simulink library "ESTS_FRIC"  (R2024b)
settings: Solver=VariableStepAuto  StartTime=0.0  StopTime=10.0  RelTol=1e-3
libraries: ESTS_FRIC_HILO x1, ESTS_FRIC_SLIP x1
settings Model: Creator=blatak  LastModifiedBy=blatak
settings ModelReferenceCC: EnableRefExpFcnMdlSchedulingChecks=on
settings RTWCC: GPUComputeCapability=3.5

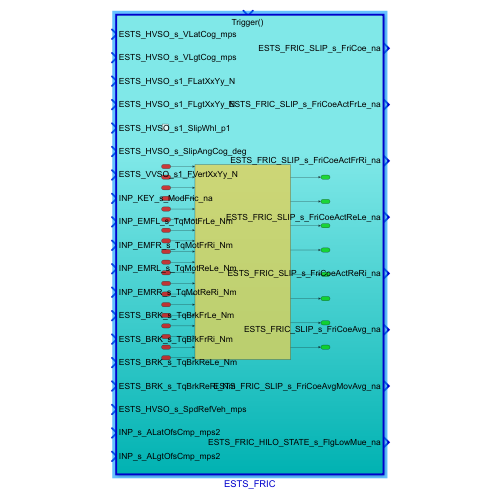
[thumbnail: Simulink's stored preview of the top-level diagram]
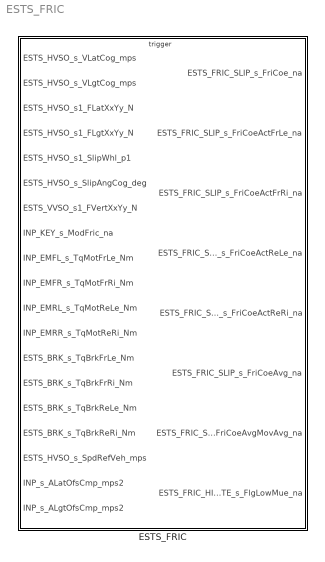
== system ESTS_FRIC ==
  ESTS_FRIC : Subsystem

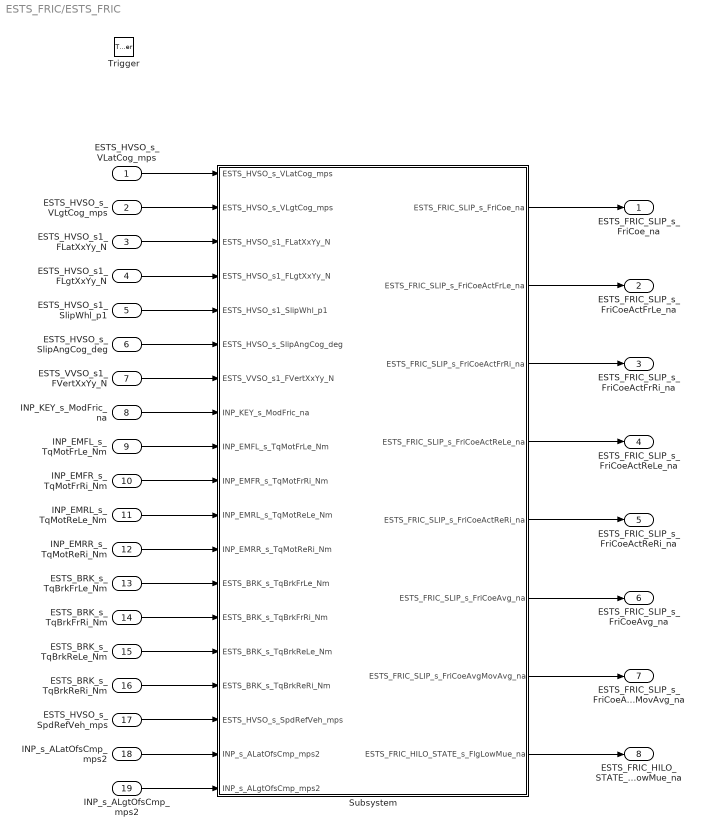
== system ESTS_FRIC/ESTS_FRIC ==
  ESTS_HVSO_s_VLatCog_mps : Inport
  ESTS_HVSO_s_VLgtCog_mps : Inport  Port=2
  ESTS_HVSO_s1_FLatXxYy_N : Inport  Port=3
  ESTS_HVSO_s1_FLgtXxYy_N : Inport  Port=4
  ESTS_HVSO_s1_SlipWhl_p1 : Inport  Port=5
  ESTS_HVSO_s_SlipAngCog_deg : Inport  Port=6
  ESTS_VVSO_s1_FVertXxYy_N : Inport  Port=7
  INP_KEY_s_ModFric_na : Inport  Port=8
  INP_EMFL_s_TqMotFrLe_Nm : Inport  Port=9
  INP_EMFR_s_TqMotFrRi_Nm : Inport  Port=10
  INP_EMRL_s_TqMotReLe_Nm : Inport  Port=11
  INP_EMRR_s_TqMotReRi_Nm : Inport  Port=12
  ESTS_BRK_s_TqBrkFrLe_Nm : Inport  Port=13
  ESTS_BRK_s_TqBrkFrRi_Nm : Inport  Port=14
  ESTS_BRK_s_TqBrkReLe_Nm : Inport  Port=15
  ESTS_BRK_s_TqBrkReRi_Nm : Inport  Port=16
  ESTS_HVSO_s_SpdRefVeh_mps : Inport  Port=17
  INP_s_ALatOfsCmp_mps2 : Inport  Port=18
  INP_s_ALgtOfsCmp_mps2 : Inport  Port=19
  Trigger : TriggerPort  TriggerType=function-call  VariantControl=(inherit)  PortDimensions=1
  Subsystem : Subsystem
  ESTS_FRIC_SLIP_s_FriCoe_na : Outport
  ESTS_FRIC_SLIP_s_FriCoeActFrLe_na : Outport  Port=2
  ESTS_FRIC_SLIP_s_FriCoeActFrRi_na : Outport  Port=3
  ESTS_FRIC_SLIP_s_FriCoeActReLe_na : Outport  Port=4
  ESTS_FRIC_SLIP_s_FriCoeActReRi_na : Outport  Port=5
  ESTS_FRIC_SLIP_s_FriCoeAvg_na : Outport  Port=6
  ESTS_FRIC_SLIP_s_FriCoeAvgMovAvg_na : Outport  Port=7
  ESTS_FRIC_HILO_STATE_s_FlgLowMue_na : Outport  Port=8
  wires:
  Subsystem/1(ESTS_FRIC_SLIP_s_FriCoe_na) -> ESTS_FRIC_SLIP_s_FriCoe_na/1
  Subsystem/2(ESTS_FRIC_SLIP_s_FriCoeActFrLe_na) -> ESTS_FRIC_SLIP_s_FriCoeActFrLe_na/1
  Subsystem/3(ESTS_FRIC_SLIP_s_FriCoeActFrRi_na) -> ESTS_FRIC_SLIP_s_FriCoeActFrRi_na/1
  Subsystem/4(ESTS_FRIC_SLIP_s_FriCoeActReLe_na) -> ESTS_FRIC_SLIP_s_FriCoeActReLe_na/1
  Subsystem/5(ESTS_FRIC_SLIP_s_FriCoeActReRi_na) -> ESTS_FRIC_SLIP_s_FriCoeActReRi_na/1
  Subsystem/6(ESTS_FRIC_SLIP_s_FriCoeAvg_na) -> ESTS_FRIC_SLIP_s_FriCoeAvg_na/1
  Subsystem/7(ESTS_FRIC_SLIP_s_FriCoeAvgMovAvg_na) -> ESTS_FRIC_SLIP_s_FriCoeAvgMovAvg_na/1
  Subsystem/8(ESTS_FRIC_HILO_STATE_s_FlgLowMue_na) -> ESTS_FRIC_HILO_STATE_s_FlgLowMue_na/1
  ESTS_HVSO_s_VLatCog_mps/1 -> Subsystem/1(ESTS_HVSO_s_VLatCog_mps)
  ESTS_HVSO_s_VLgtCog_mps/1 -> Subsystem/2(ESTS_HVSO_s_VLgtCog_mps)
  ESTS_HVSO_s1_FLatXxYy_N/1 -> Subsystem/3(ESTS_HVSO_s1_FLatXxYy_N)
  ESTS_HVSO_s1_FLgtXxYy_N/1 -> Subsystem/4(ESTS_HVSO_s1_FLgtXxYy_N)
  ESTS_HVSO_s1_SlipWhl_p1/1 -> Subsystem/5(ESTS_HVSO_s1_SlipWhl_p1)
  ESTS_HVSO_s_SlipAngCog_deg/1 -> Subsystem/6(ESTS_HVSO_s_SlipAngCog_deg)
  ESTS_VVSO_s1_FVertXxYy_N/1 -> Subsystem/7(ESTS_VVSO_s1_FVertXxYy_N)
  INP_KEY_s_ModFric_na/1 -> Subsystem/8(INP_KEY_s_ModFric_na)
  INP_EMFL_s_TqMotFrLe_Nm/1 -> Subsystem/9(INP_EMFL_s_TqMotFrLe_Nm)
  INP_EMFR_s_TqMotFrRi_Nm/1 -> Subsystem/10(INP_EMFR_s_TqMotFrRi_Nm)
  INP_EMRL_s_TqMotReLe_Nm/1 -> Subsystem/11(INP_EMRL_s_TqMotReLe_Nm)
  INP_EMRR_s_TqMotReRi_Nm/1 -> Subsystem/12(INP_EMRR_s_TqMotReRi_Nm)
  ESTS_BRK_s_TqBrkFrLe_Nm/1 -> Subsystem/13(ESTS_BRK_s_TqBrkFrLe_Nm)
  ESTS_BRK_s_TqBrkFrRi_Nm/1 -> Subsystem/14(ESTS_BRK_s_TqBrkFrRi_Nm)
  ESTS_BRK_s_TqBrkReLe_Nm/1 -> Subsystem/15(ESTS_BRK_s_TqBrkReLe_Nm)
  ESTS_BRK_s_TqBrkReRi_Nm/1 -> Subsystem/16(ESTS_BRK_s_TqBrkReRi_Nm)
  ESTS_HVSO_s_SpdRefVeh_mps/1 -> Subsystem/17(ESTS_HVSO_s_SpdRefVeh_mps)
  INP_s_ALatOfsCmp_mps2/1 -> Subsystem/18(INP_s_ALatOfsCmp_mps2)
  INP_s_ALgtOfsCmp_mps2/1 -> Subsystem/19(INP_s_ALgtOfsCmp_mps2)

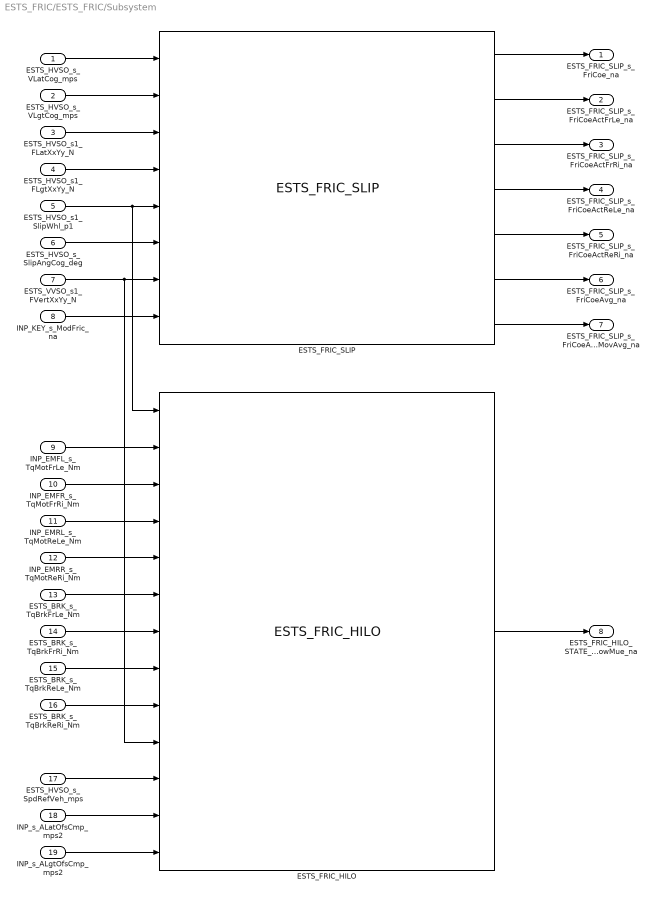
== system ESTS_FRIC/ESTS_FRIC/Subsystem ==
  ESTS_HVSO_s_VLatCog_mps : Inport
  ESTS_HVSO_s_VLgtCog_mps : Inport  Port=2
  ESTS_HVSO_s1_FLatXxYy_N : Inport  Port=3
  ESTS_HVSO_s1_FLgtXxYy_N : Inport  Port=4
  ESTS_HVSO_s1_SlipWhl_p1 : Inport  Port=5
  ESTS_HVSO_s_SlipAngCog_deg : Inport  Port=6
  ESTS_VVSO_s1_FVertXxYy_N : Inport  Port=7
  INP_KEY_s_ModFric_na : Inport  Port=8
  INP_EMFL_s_TqMotFrLe_Nm : Inport  Port=9
  INP_EMFR_s_TqMotFrRi_Nm : Inport  Port=10
  INP_EMRL_s_TqMotReLe_Nm : Inport  Port=11
  INP_EMRR_s_TqMotReRi_Nm : Inport  Port=12
  ESTS_BRK_s_TqBrkFrLe_Nm : Inport  Port=13
  ESTS_BRK_s_TqBrkFrRi_Nm : Inport  Port=14
  ESTS_BRK_s_TqBrkReLe_Nm : Inport  Port=15
  ESTS_BRK_s_TqBrkReRi_Nm : Inport  Port=16
  ESTS_HVSO_s_SpdRefVeh_mps : Inport  Port=17
  INP_s_ALatOfsCmp_mps2 : Inport  Port=18
  INP_s_ALgtOfsCmp_mps2 : Inport  Port=19
  ESTS_FRIC_HILO : ESTS_FRIC_HILO/ESTS_FRIC_HILO  SystemSampleTime=-1  VariantActivationTime=update diagram  AllowFlexibleInterface=on  Latency=0  AutoFrameSizeCalculation=off
  ESTS_FRIC_SLIP : ESTS_FRIC_SLIP/ESTS_FRIC_SLIP  SystemSampleTime=-1  VariantActivationTime=update diagram  AllowFlexibleInterface=on  Latency=0  AutoFrameSizeCalculation=off
  ESTS_FRIC_SLIP_s_FriCoe_na : Outport
  ESTS_FRIC_SLIP_s_FriCoeActFrLe_na : Outport  Port=2
  ESTS_FRIC_SLIP_s_FriCoeActFrRi_na : Outport  Port=3
  ESTS_FRIC_SLIP_s_FriCoeActReLe_na : Outport  Port=4
  ESTS_FRIC_SLIP_s_FriCoeActReRi_na : Outport  Port=5
  ESTS_FRIC_SLIP_s_FriCoeAvg_na : Outport  Port=6
  ESTS_FRIC_SLIP_s_FriCoeAvgMovAvg_na : Outport  Port=7
  ESTS_FRIC_HILO_STATE_s_FlgLowMue_na : Outport  Port=8
  wires:
  ESTS_HVSO_s_VLatCog_mps/1 -> ESTS_FRIC_SLIP/1
  ESTS_HVSO_s_VLgtCog_mps/1 -> ESTS_FRIC_SLIP/2
  ESTS_HVSO_s1_FLatXxYy_N/1 -> ESTS_FRIC_SLIP/3
  ESTS_HVSO_s1_FLgtXxYy_N/1 -> ESTS_FRIC_SLIP/4
  ESTS_HVSO_s1_SlipWhl_p1/1 -> ESTS_FRIC_HILO/1, ESTS_FRIC_SLIP/5
  ESTS_HVSO_s_SlipAngCog_deg/1 -> ESTS_FRIC_SLIP/6
  ESTS_VVSO_s1_FVertXxYy_N/1 -> ESTS_FRIC_HILO/10, ESTS_FRIC_SLIP/7
  INP_KEY_s_ModFric_na/1 -> ESTS_FRIC_SLIP/8
  INP_EMFL_s_TqMotFrLe_Nm/1 -> ESTS_FRIC_HILO/2
  INP_EMFR_s_TqMotFrRi_Nm/1 -> ESTS_FRIC_HILO/3
  INP_EMRL_s_TqMotReLe_Nm/1 -> ESTS_FRIC_HILO/4
  INP_EMRR_s_TqMotReRi_Nm/1 -> ESTS_FRIC_HILO/5
  ESTS_BRK_s_TqBrkFrLe_Nm/1 -> ESTS_FRIC_HILO/6
  ESTS_BRK_s_TqBrkFrRi_Nm/1 -> ESTS_FRIC_HILO/7
  ESTS_BRK_s_TqBrkReLe_Nm/1 -> ESTS_FRIC_HILO/8
  ESTS_BRK_s_TqBrkReRi_Nm/1 -> ESTS_FRIC_HILO/9
  ESTS_HVSO_s_SpdRefVeh_mps/1 -> ESTS_FRIC_HILO/11
  INP_s_ALatOfsCmp_mps2/1 -> ESTS_FRIC_HILO/12
  INP_s_ALgtOfsCmp_mps2/1 -> ESTS_FRIC_HILO/13
  ESTS_FRIC_SLIP/1 -> ESTS_FRIC_SLIP_s_FriCoe_na/1
  ESTS_FRIC_SLIP/2 -> ESTS_FRIC_SLIP_s_FriCoeActFrLe_na/1
  ESTS_FRIC_SLIP/3 -> ESTS_FRIC_SLIP_s_FriCoeActFrRi_na/1
  ESTS_FRIC_SLIP/4 -> ESTS_FRIC_SLIP_s_FriCoeActReLe_na/1
  ESTS_FRIC_SLIP/5 -> ESTS_FRIC_SLIP_s_FriCoeActReRi_na/1
  ESTS_FRIC_SLIP/6 -> ESTS_FRIC_SLIP_s_FriCoeAvg_na/1
  ESTS_FRIC_SLIP/7 -> ESTS_FRIC_SLIP_s_FriCoeAvgMovAvg_na/1
  ESTS_FRIC_HILO/1 -> ESTS_FRIC_HILO_STATE_s_FlgLowMue_na/1
